simulink model "test_image"  (R2023a)
settings: Solver=VariableStepAuto  StartTime=0.0  StopTime=5  RelTol=1e-3
libraries: visionsinks x3, visionmorphops x2, visionstatistics x1, visionsources x1
settings Model: Creator=avizinho  LastModifiedBy=avizinho

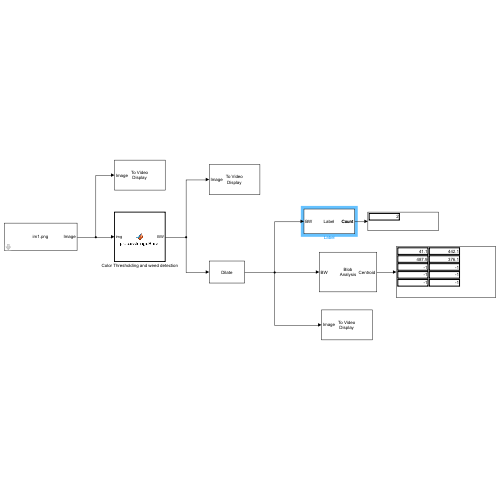
[thumbnail: Simulink's stored preview of the top-level diagram]
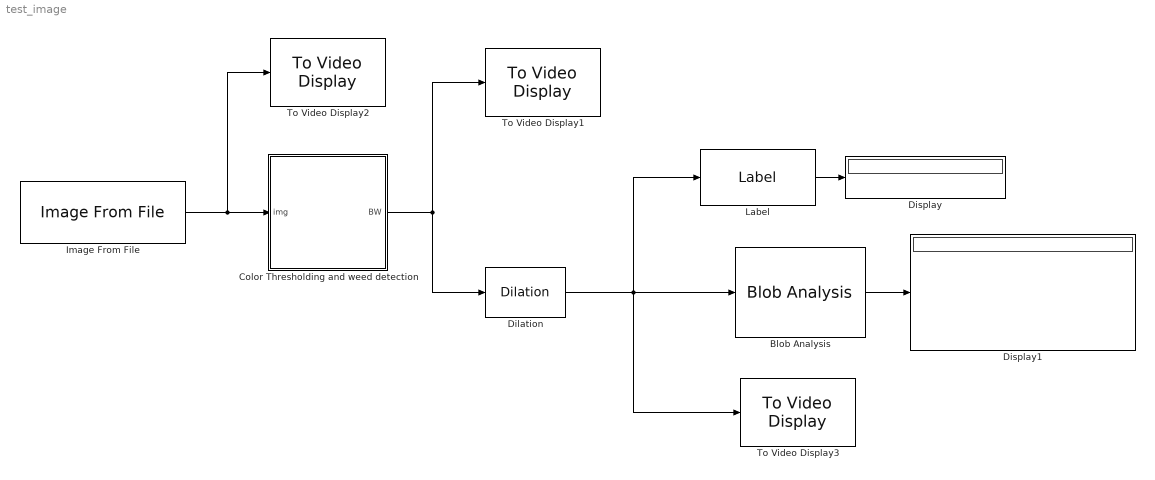
== system test_image ==
  Blob Analysis : visionstatistics/Blob Analysis  Tag=vipblks_row_conv  area=off  centroid=on  bBox=off  majorAxis=off  minorAxis=off  angle=off  eccentricity=off  equivDiameterSq=off  extent=off  perimeter=off  outDT=double  conn=8  isLabel=off  maxBlobs=5  warnIfNumBlobsExceeded=on  isCount=off  useMinArea=off  minArea=300  useMaxArea=off  maxArea=intmax('uint32')  excludeBorderBlob=off  isOutVarDim=off  isFill=on  fillValues=-1  roundingMode=Floor  overflowMode=off  prodOutputMode=Binary point scaling  prodOutputWordLength=32  prodOutputFracLength=16  accumMode=Binary point scaling  accumWordLength=32  accumFracLength=0  outputMode=Binary point scaling  outputWordLength=32  outputFracLength=16  firstCoeffMode=Binary point scaling  firstCoeffWordLength=16  firstCoeffFracLength=14  secondCoeffMode=Binary point scaling  secondCoeffWordLength=32  secondCoeffFracLength=16
  Color Thresholding and weed detection : MATLAB Function  TreatAsAtomicUnit=on  VariantControl=Basic
  Dilation : visionmorphops/Dilation  nhoodsrc=Specify via dialog  strel=ones(10,10)
  Display : Display
  Display1 : Display
  Image From File : visionsources/Image From File  Tag=vipblks_nd  FileName=C:\work\PASS\PARC\2023\test_publisher\scripts\im1.png  Ts=0.5  imagePorts=One multidimensional signal  OutPortLabels=R|G|B  ImageDataType=Inherit from input image  sdImageDataType=uint(8)  Signed=on  WordLength=16  FractionLengthMode=User-defined  FractionLength=15
  Label : visionmorphops/Label  conn=8  output=Number of labels  outType=Automatic  lastLabel=maximum value of the output data type
  To Video Display1 : visionsinks/To Video Display  windowSizeMode=Normal  openAtMdlStart=on  fullScreen=off  videoWindowX=689  videoWindowY=179  saveWindowSize=off  videoWindowWidth=640  videoWindowHeight=480  inputColorFormat=RGB  inputType=Obsolete  imagePorts=One multidimensional signal  OutputDevice=On-screen video monitor  dataOrg=Column-major  isWindowOpen=off
  To Video Display2 : visionsinks/To Video Display  windowSizeMode=Normal  openAtMdlStart=on  fullScreen=off  videoWindowX=53  videoWindowY=180  saveWindowSize=off  videoWindowWidth=640  videoWindowHeight=480  inputColorFormat=RGB  inputType=Obsolete  imagePorts=One multidimensional signal  OutputDevice=On-screen video monitor  dataOrg=Column-major  isWindowOpen=off
  To Video Display3 : visionsinks/To Video Display  windowSizeMode=Normal  openAtMdlStart=on  fullScreen=off  videoWindowX=1226  videoWindowY=183  saveWindowSize=off  videoWindowWidth=643  videoWindowHeight=477  inputColorFormat=RGB  inputType=Obsolete  imagePorts=One multidimensional signal  OutputDevice=On-screen video monitor  dataOrg=Column-major  isWindowOpen=off
  wires:
  Image From File/1 -> To Video Display2/1, Color Thresholding and weed detection/1(img)
  Label/1 -> Display/1
  Blob Analysis/1 -> Display1/1
  Dilation/1 -> To Video Display3/1, Label/1, Blob Analysis/1
  Color Thresholding and weed detection/1(BW) -> Dilation/1, To Video Display1/1

== matlab function test_image/Color Thresholding and weed detection ==
  data: img input; BW output
function BW= processImageBasic(img)

% Convert RGB image to chosen color space
I = rgb2lab(img);

% Define thresholds for channel 1 based on histogram settings
channel1Min = 27.074;
channel1Max = 87.009;

% Define thresholds for channel 2 based on histogram settings
channel2Min = -21.242;
channel2Max = -7.642;

% Define thresholds for channel 3 based on histogram settings
channel3Min = 40.393;
channel3Max = 59.976;

% Create mask based on chosen histogram thresholds
sliderBW = (I(:,:,1) >= channel1Min ) & (I(:,:,1) <= channel1Max) & ...
    (I(:,:,2) >= channel2Min ) & (I(:,:,2) <= channel2Max) & ...
    (I(:,:,3) >= channel3Min ) & (I(:,:,3) <= channel3Max);
BW = sliderBW;
BW=bwareaopen(BW, 50);

end
